simulink model "SingleTrackCANoe"  (R2021b)
settings: Solver=ode1  StartTime=0  StopTime=2  FixedStep=1.0000000000000000e-003  RelTol=1e-3
InitFcn:
  | sampleTime = str2double(get_param(bdroot, 'FixedStep'));
undefined symbols (not defined in the file or in its folder): AccPedalPos, BrakePedalPos, BrakeSwitch, DiscIntNeverNeededParam, DYNA4, EngSpd, IgnitionSwitch, InitialGear, InitialSpeed, IntendedEngTrq, LeftIndicator, MainBrakePress, MaxGear, MDL, MinGear, RefAcc, RefLane, RefLatPos, RefPath, RefPathCurv, RefSpd, RefSpdPreview, RefSpdRetrospect, RightIndicator, SteeringWheelAng, SteeringWheelTrq, UserDefinedRefValue, vm_const
libraries: UtilitiesLibrary x62, simulink x18, WheelSystemModules x14, LongitudinalControllerModules x13, LateralControllerModules x7, AnimationBusselectorModules x5, EnvironmentModules x5, BasicEngineControlModules x5, MiscellaneousControlModules x5, Animation3Modules x4, AuxiliariesModules x4, ReducedTireModules x4
(part 12 of 34)

== system SingleTrackCANoe/SimulationModel/Vehicle/Engine/EngineControlUnit ==
  fromEnginePhysics : Inport
  fromCTRL : Inport  Port=2
  fromEnvironment : Inport  Port=3
  fromChassis : Inport  Port=4
  fromDrivetrain : Inport  Port=5
  fromElectricalSystem : Inport  Port=6
  ASR/MSR : BasicEngineControlModules/ASR//MSR  SystemSampleTime=-1  VariantActivationTime=update diagram  Latency=0  AutoFrameSizeCalculation=off
  Data Type Conversion{,1..4} (5 alike) : DataTypeConversion  OutDataTypeStr=double
  DynaComponentInfo : Subsystem  Tag=DynaComponentInfo
      mask init:
      | data= get_param(gcb, 'UserData');
      settings: OpenFcn=DYNA4.ModelHandling.Component.ShowEditComponentInformationDialog(gcb);
      mask Display: disp(['Type = ', data.type, '\nGroup = ', data.group, '\nName = ', data.name ])
  EngineControlUnitOutput : Subsystem  Tag=TESIS DYNAware Interface Block  mask{NeedsUpdate=off, SignalInfo=|}
      mask SignalInfo=|
      | {
      |   "Version": "4.6",
      |   "MuxedOutputBusName": "EngineControlUnit",
      |   "MuxedInputBusName": "input",
      |   "MuxedInputSelected": false,
      |   "MuxedOutputSelected": true,
      |   "SignalData": [
      |     {
      |       "initialValue": "0.0",
      |       "name": "StarterSwitch[0;1]",
      |       "comment": "Engine starter switch",
      |       "minString": "",
      |       "maxString": "",
      |       "width": 1,
      |       "dataType": 0,
      |       "signalType": 0,
      |       "createSignal": false,
      |       "outputName": "StarterSwitch[0;1]",
      |       "generateSignalAccessBlock": false,
      |       "accessId": "$(parentId).$(blockName).$(outputName)"
      |     },
      |     {
      |       "initialValue": "0.0",
      |       "name": "EngRunPermission[0;1]",
      |       "comment": "Switch indicating a engine stop due to start stop function or ignition off",
      |       "minString": "",
      |       "maxString": "",
      |       "width": 1,
      |       "dataType": 0,
      |       "signalType": 0,
      |       "createSignal": false,
      |       "outputName": "EngRunPermission[0;1]",
      |       "generateSignalAccessBlock": false,
      |       "accessId": "$(parentId).$(blockName).$(outputName)"
      |     },
      |     {
      |       "initialValue": "0.0",
      |       "name": "EngLoadSignal[0_1]",
      |       "comment": "Engine load signal",
      |       "minString": "",
      |       "maxString": "",
      |       "width": 1,
      |       "dataType": 0,
      |       "signalType": 0,
      |       "createSignal": false,
      |       "outputName": "EngLoadSignal[0_1]",
      |       "generateSignalAccessBlock": false,
      |       "accessId": "$(parentId).$(blockName).$(outputName)"
      |     },
      |     {
      |       "initialValue": "0.0",
      |       "name": "EngIdleSpd[rad/s]",
      |       "comment": "Engine idle speed",
      |       "minString": "",
      |       "maxString": "",
      |       "width": 1,
      |       "dataType": 0,
      |       "signalType": 0,
      |       "createSignal": false,
      |       "outputName": "EngIdleSpd[rad/s]",
      |       "generateSignalAccessBlock": false,
      |       "accessId": "$(parentId).$(blockName).$(outputName)"
      |     },
      |     {
      |       "initialValue": "0.0",
      |       "name": "EngFuelCutoff[0;1]",
      |       "comment": "Logical signal which is true if fuel mass flow is stopped",
      |       "minString": "",
      |       "maxString": "",
      |       "width": 1,
      |       "dataType": 0,
      |       "signalType": 0,
      |       "createSignal": false,
      |       "outputName": "EngFuelCutoff[0;1]",
      |       "generateSignalAccessBlock": false,
      |       "accessId": "$(parentId).$(blockName).$(outputName)"
      |     },
      |     {
      |       "initialValue": "0.0",
      |       "name": "MaxEngSpd[rad/s]",
      |       "comment": "Maximum allowed engine speed, threshold for fuel cut off",
      |       "minString": "",
      |       "maxString": "",
      |       "width": 1,
      |       "dataType": 0,
      |       "signalType": 0,
      |       "createSignal": false,
      |       "outputName": "MaxEngSpd[rad/s]",
      |       "generateSignalAccessBlock": false,
      |       "accessId": "$(parentId).$(blockName).$(outputName)"
      |     },
      |     {
      |       "initialValue": "0.0",
      |       "name": "UpperEngTrqSwitch[0;2]",
      |       "comment": "Switch indicating how the upper engine torque should be restricted (0: off, 1: slow, 2: fast)",
      |       "minString": "",
      |       "maxString": "",
      |       "width": 1,
      |       "dataType": 0,
      |       "signalType": 0,
      |       "createSignal": false,
      |       "outputName": "UpperEngTrqSwitch[0;2]",
      |       "generateSignalAccessBlock": false,
      |       "accessId": "$(parentId).$(blockName).$(outputName)"
      |     },
      |     {
      |       "initialValue": "0.0",
      |       "name": "UpperEngTrqLimit[Nm]",
      |       "comment": "Upper limit for the engine torque",
      |       "minString": "",
      |       "maxString": "",
      |       "width": 1,
      |       "dataType": 0,
      |       "signalType": 0,
      |       "createSignal": false,
      |       "outputName": "UpperEngTrqLimit[Nm]",
      |       "generateSignalAccessBlock": false,
      |       "accessId": "$(parentId).$(blockName).$(outputName)"
      |     },
      |     {
      |       "initialValue": "0.0",
      |       "name": "LowerEngTrqSwitch[0;2]",
      |       "comment": "Switch indicating how the lower engine torque should be restricted (0: off, 1: slow, 2: fast)",
      |       "minString": "",
      |       "maxString": "",
      |       "width": 1,
      |       "dataType": 0,
      |       "signalType": 0,
      |       "createSignal": false,
      |       "outputName": "LowerEngTrqSwitch[0;2]",
      |       "generateSignalAccessBlock": false,
      |       "accessId": "$(parentId).$(blockName).$(outputName)"
      |     },
      |     {
      |       "initialValue": "0.0",
      |       "name": "LowerEngTrqLimit[Nm]",
      |       "comment": "Lower limit for the engine torque",
      |       "minString": "",
      |       "maxString": "",
      |       "width": 1,
      |       "dataType": 0,
      |       "signalType": 0,
      |       "createSignal": false,
      |       "outputName": "LowerEngTrqLimit[Nm]",
      |       "generateSignalAccessBlock": false,
      |       "accessId": "$(parentId).$(blockName).$(outputName)"
      |     }
      |   ]
      | }
      mask prompts: NeedsUpdate "Specify, if subsystem content needs to be updated"; SignalInfo "Signal Info (json)"
      mask help: DYNA4 Interface Block Version 4.6
      mask init:
      | blockName = get_param(gcbh, 'Name');
      | parentId = DYNA4.ModelHandling.AccessID.getFromHierarchy(gcbh);
      | TD.InterfaceBlock.ModelCallbacks.GenerateContent(gcb);
      settings: DeleteFcn=TD.InterfaceBlock.ModelCallbacks.CloseGUI( gcbh );  NameChangeFcn=TD.InterfaceBlock.ModelCallbacks.BlockRenamedHandler(gcbh);  OpenFcn=TD.InterfaceBlock.ModelCallbacks.OpenGUI( gcbh );  CloseFcn=TD.InterfaceBlock.ModelCallbacks.CloseGUI( gcbh );
      mask Display:
      | image('InterfaceBlock.png','center');
      | port_label('input',1, 'StarterSwitch[0;1]');
      | port_label('input',2, 'EngRunPermission[0;1]');
      | port_label('input',3, 'EngLoadSignal[0_1]');
      | port_label('input',4, 'EngIdleSpd[rad/s]');
      | port_label('input',5, 'EngFuelCutoff[0;1]');
      | port_label('input',6, 'MaxEngSpd[rad/s]');
      | port_label('input',7, 'UpperEngTrqSwitch[0;2]');
      | port_label('input',8, 'UpperEngTrqLimit[Nm]');
      | port_label('input',9, 'LowerEngTrqSwitch[0;2]');
      | port_label('input',10, 'LowerEngTrqLimit[Nm]');
      | port_label('output',1, 'EngineControlUnit');
  EngineStartStopLogic : BasicEngineControlModules/EngineStartStopLogic  SystemSampleTime=-1  VariantActivationTime=update diagram  Latency=0  AutoFrameSizeCalculation=off
  FuelCutoff : BasicEngineControlModules/FuelCutoff  DATA_NODE=MDL.Vehicle.Engine.EngineControlUnit.FuelCutoff  FuelCutoffTimeConst=MDL.Vehicle.Engine.EngineControlUnit.FuelCutoff.FuelCutoffTimeConst  FuelCutoffPedalMax=MDL.Vehicle.Engine.EngineControlUnit.FuelCutoff.FuelCutoffMaxLoadSig  MaxEngSpd=MDL.Vehicle.Engine.EngineControlUnit.FuelCutoff.MaxEngSpd
  IdleSpeedController : BasicEngineControlModules/IdleSpeedController  DATA_NODE=MDL.Vehicle.Engine.EngineControlUnit.IdleSpeedController  RefEngIdleSpd=MDL.Vehicle.Engine.EngineControlUnit.IdleSpeedController.RefEngIdleSpd  UpperIdleSpeedThreshold=MDL.Vehicle.Engine.EngineControlUnit.IdleSpeedController.UpperIdleSpdThres  LowerIdleSpeedThreshold=MDL.Vehicle.Engine.EngineControlUnit.IdleSpeedController.LowerIdleSpdThres  MaxCtrlTrq=MDL.Vehicle.Engine.EngineControlUnit.IdleSpeedController.MaxIdleSpdRefTrq  MinCtrlTrq=MDL.Vehicle.Engine.EngineControlUnit.IdleSpeedController.MinIdleSpdRefTrq  IdleCtl_P=MDL.Vehicle.Engine.EngineControlUnit.IdleSpeedController.ProportionalGain  IdleCtl_I=MDL.Vehicle.Engine.EngineControlUnit.IdleSpeedController.IntegralGain  IdleCtl_D=MDL.Vehicle.Engine.EngineControlUnit.IdleSpeedController.DerivativeGain  IdleCtl_N=MDL.Vehicle.Engine.EngineControlUnit.IdleSpeedController.DerivativeFilterCutoffFreq  MaxIgnitionOffsetAng=MDL.Vehicle.Engine.EngineControlUnit.IdleSpeedController.MaxIgnitionOffsetAng  IgnitionDelayReductionTrq=MDL.Vehicle.Engine.EngineControlUnit.IdleSpeedController.IgnitionDelayReductionTrq  IntendedEngineStartTime=MDL.Vehicle.Engine.EngineControlUnit.IdleSpeedController.IntendedEngineStartTime
  InputFromCTRL : Subsystem  Tag=TESIS DYNAware Interface Block  mask{NeedsUpdate=off, SignalInfo=|}
      mask SignalInfo=|
      | {
      |   "Version": "4.6",
      |   "MuxedOutputBusName": "Drivetrain",
      |   "MuxedInputBusName": "fromCTRL",
      |   "MuxedInputSelected": true,
      |   "MuxedOutputSelected": false,
      |   "SignalData": [
      |     {
      |       "initialValue": "0.0",
      |       "name": "CTRL.LongitudinalControl.IgnitionSwitch[0;3]",
      |       "comment": "Ignition signal with four signal states: 0 - ignition off + consumer off + starter off, 1 - ignition off + consumer on + starter off, 2 - ignition on + consumer on + starter off, 3 - ignition on + consumer on  + starter on",
      |       "minString": "",
      |       "maxString": "",
      |       "width": 1,
      |       "dataType": 0,
      |       "signalType": 0,
      |       "createSignal": false,
      |       "outputName": "IgnitionSwitch[0;3]",
      |       "generateSignalAccessBlock": false,
      |       "accessId": "$(parentId).$(blockName).$(outputName)"
      |     },
      |     {
      |       "initialValue": "0.0",
      |       "name": "CTRL.LongitudinalControl.EngRunPermission[0;1]",
      |       "comment": "",
      |       "minString": "",
      |       "maxString": "",
      |       "width": 1,
      |       "dataType": 0,
      |       "signalType": 0,
      |       "createSignal": false,
      |       "outputName": "EngRunPermission[0;1]",
      |       "generateSignalAccessBlock": false,
      |       "accessId": "$(parentId).$(blockName).$(outputName)"
      |     },
      |     {
      |       "initialValue": "0.0",
      |       "name": "CTRL.LongitudinalControl.AccPedalPos[0_1]",
      |       "comment": "",
      |       "minString": "",
      |       "maxString": "",
      |       "width": -1,
      |       "dataType": 0,
      |       "signalType": 0,
      |       "createSignal": false,
      |       "outputName": "AccPedalPos[0_1]",
      |       "generateSignalAccessBlock": false,
      |       "accessId": "$(parentId).$(blockName).$(outputName)"
      |     },
      |     {
      |       "initialValue": "0.0",
      |       "name": "CTRL.LongitudinalControl.IntendedEngTrq[Nm]",
      |       "comment": "",
      |       "minString": "",
      |       "maxString": "",
      |       "width": 1,
      |       "dataType": 0,
      |       "signalType": 0,
      |       "createSignal": false,
      |       "outputName": "IntendedEngTrq[Nm]",
      |       "generateSignalAccessBlock": false,
      |       "accessId": "$(parentId).$(blockName).$(outputName)"
      |     },
      |     {
      |       "initialValue": "0.0",
      |       "name": "CTRL.LongitudinalControl.IntendedEngTrqActive[0;1]",
      |       "comment": "",
      |       "minString": "",
      |       "maxString": "",
      |       "width": 1,
      |       "dataType": 0,
      |       "signalType": 0,
      |       "createSignal": false,
      |       "outputName": "IntendedEngTrqActive[0;1]",
      |       "generateSignalAccessBlock": false,
      |       "accessId": "$(parentId).$(blockName).$(outputName)"
      |     },
      |     {
      |       "initialValue": "0.0",
      |       "name": "CTRL.LongitudinalControl.ClutchPos[0_1]",
      |       "comment": "Clutch position",
      |       "minString": "",
      |       "maxString": "",
      |       "width": 1,
      |       "dataType": 0,
      |       "signalType": 0,
      |       "createSignal": false,
      |       "outputName": "ClutchPos[0_1]",
      |       "generateSignalAccessBlock": false,
      |       "accessId": "$(parentId).$(blockName).$(outputName)"
      |     }
      |   ]
      | }
      mask prompts: NeedsUpdate "Specify, if subsystem content needs to be updated"; SignalInfo "Signal Info (json)"
      mask help: DYNA4 Interface Block Version 4.6
      mask init:
      | blockName = get_param(gcbh, 'Name');
      | parentId = DYNA4.ModelHandling.AccessID.getFromHierarchy(gcbh);
      | TD.InterfaceBlock.ModelCallbacks.GenerateContent(gcb);
      settings: DeleteFcn=TD.InterfaceBlock.ModelCallbacks.CloseGUI( gcbh );  NameChangeFcn=TD.InterfaceBlock.ModelCallbacks.BlockRenamedHandler(gcbh);  OpenFcn=TD.InterfaceBlock.ModelCallbacks.OpenGUI( gcbh );  CloseFcn=TD.InterfaceBlock.ModelCallbacks.CloseGUI( gcbh );
      mask Display:
      | image('InterfaceBlock.png','center');
      | port_label('input',1, 'fromCTRL');
      | port_label('output',1, 'IgnitionSwitch[0;3]');
      | port_label('output',2, 'EngRunPermission[0;1]');
      | port_label('output',3, 'AccPedalPos[0_1]');
      | port_label('output',4, 'IntendedEngTrq[Nm]');
      | port_label('output',5, 'IntendedEngTrqActive[0;1]');
      | port_label('output',6, 'ClutchPos[0_1]');
  InputFromCTRL1 : Subsystem  Tag=TESIS DYNAware Interface Block  mask{NeedsUpdate=off, SignalInfo=|}
      mask SignalInfo=|
      | {
      |   "Version": "4.6",
      |   "MuxedOutputBusName": "Drivetrain",
      |   "MuxedInputBusName": "fromCTRL",
      |   "MuxedInputSelected": true,
      |   "MuxedOutputSelected": false,
      |   "SignalData": [
      |     {
      |       "initialValue": "0.0",
      |       "name": "CTRL.LongitudinalControl.ASRRequestSwitch[0;2]",
      |       "comment": "",
      |       "minString": "",
      |       "maxString": "",
      |       "width": -1,
      |       "dataType": 0,
      |       "signalType": 0,
      |       "createSignal": false,
      |       "outputName": "ASRRequestSwitch[0;2]",
      |       "generateSignalAccessBlock": false,
      |       "accessId": "$(parentId).$(blockName).$(outputName)"
      |     },
      |     {
      |       "initialValue": "0.0",
      |       "name": "CTRL.LongitudinalControl.ASRTrq[Nm]",
      |       "comment": "",
      |       "minString": "",
      |       "maxString": "",
      |       "width": -1,
      |       "dataType": 0,
      |       "signalType": 0,
      |       "createSignal": false,
      |       "outputName": "ASRTrq[Nm]",
      |       "generateSignalAccessBlock": false,
      |       "accessId": "$(parentId).$(blockName).$(outputName)"
      |     },
      |     {
      |       "initialValue": "0.0",
      |       "name": "CTRL.LongitudinalControl.MSRRequestSwitch[0;2]",
      |       "comment": "",
      |       "minString": "",
      |       "maxString": "",
      |       "width": -1,
      |       "dataType": 0,
      |       "signalType": 0,
      |       "createSignal": false,
      |       "outputName": "MSRRequestSwitch[0;2]",
      |       "generateSignalAccessBlock": false,
      |       "accessId": "$(parentId).$(blockName).$(outputName)"
      |     },
      |     {
      |       "initialValue": "0.0",
      |       "name": "CTRL.LongitudinalControl.MSRTrq[Nm]",
      |       "comment": "",
      |       "minString": "",
      |       "maxString": "",
      |       "width": -1,
      |       "dataType": 0,
      |       "signalType": 0,
      |       "createSignal": false,
      |       "outputName": "MSRTrq[Nm]",
      |       "generateSignalAccessBlock": false,
      |       "accessId": "$(parentId).$(blockName).$(outputName)"
      |     }
      |   ]
      | }
      mask prompts: NeedsUpdate "Specify, if subsystem content needs to be updated"; SignalInfo "Signal Info (json)"
      mask help: DYNA4 Interface Block Version 4.6
      mask init:
      | blockName = get_param(gcbh, 'Name');
      | parentId = DYNA4.ModelHandling.AccessID.getFromHierarchy(gcbh);
      | TD.InterfaceBlock.ModelCallbacks.GenerateContent(gcb);
      settings: DeleteFcn=TD.InterfaceBlock.ModelCallbacks.CloseGUI( gcbh );  NameChangeFcn=TD.InterfaceBlock.ModelCallbacks.BlockRenamedHandler(gcbh);  OpenFcn=TD.InterfaceBlock.ModelCallbacks.OpenGUI( gcbh );  CloseFcn=TD.InterfaceBlock.ModelCallbacks.CloseGUI( gcbh );
      mask Display:
      | image('InterfaceBlock.png','center');
      | port_label('input',1, 'fromCTRL');
      | port_label('output',1, 'ASRRequestSwitch[0;2]');
      | port_label('output',2, 'ASRTrq[Nm]');
      | port_label('output',3, 'MSRRequestSwitch[0;2]');
      | port_label('output',4, 'MSRTrq[Nm]');
  InputFromChassis : Subsystem  Tag=TESIS DYNAware Interface Block  mask{NeedsUpdate=off, SignalInfo=|}
      mask SignalInfo=|
      | {
      |   "Version": "4.6",
      |   "MuxedOutputBusName": "Drivetrain",
      |   "MuxedInputBusName": "fromChassis",
      |   "MuxedInputSelected": true,
      |   "MuxedOutputSelected": false,
      |   "SignalData": {
      |     "initialValue": "0.0",
      |     "name": "VehicleBody.AbsVel[m/s]",
      |     "comment": "",
      |     "minString": "",
      |     "maxString": "",
      |     "width": -1,
      |     "dataType": 0,
      |     "signalType": 0,
      |     "createSignal": false,
      |     "outputName": "AbsVel[m/s]",
      |     "generateSignalAccessBlock": false,
      |     "accessId": "$(parentId).$(blockName).$(outputName)"
      |   }
      | }
      mask prompts: NeedsUpdate "Specify, if subsystem content needs to be updated"; SignalInfo "Signal Info (json)"
      mask help: DYNA4 Interface Block Version 4.6
      mask init:
      | blockName = get_param(gcbh, 'Name');
      | parentId = DYNA4.ModelHandling.AccessID.getFromHierarchy(gcbh);
      | TD.InterfaceBlock.ModelCallbacks.GenerateContent(gcb);
      settings: DeleteFcn=TD.InterfaceBlock.ModelCallbacks.CloseGUI( gcbh );  NameChangeFcn=TD.InterfaceBlock.ModelCallbacks.BlockRenamedHandler(gcbh);  OpenFcn=TD.InterfaceBlock.ModelCallbacks.OpenGUI( gcbh );  CloseFcn=TD.InterfaceBlock.ModelCallbacks.CloseGUI( gcbh );
      mask Display:
      | image('InterfaceBlock.png','center');
      | port_label('input',1, 'fromChassis');
      | port_label('output',1, 'AbsVel[m/s]');
  InputFromDrivetrain : Subsystem  Tag=TESIS DYNAware Interface Block  mask{NeedsUpdate=off, SignalInfo=|}
      mask SignalInfo=|
      | {
      |   "Version": "4.6",
      |   "MuxedOutputBusName": "Drivetrain",
      |   "MuxedInputBusName": "fromDrivetrain",
      |   "MuxedInputSelected": true,
      |   "MuxedOutputSelected": false,
      |   "SignalData": [
      |     {
      |       "initialValue": "0.0",
      |       "name": "DrivetrainPhysics.Transmission.Gear[-4;20]",
      |       "comment": "",
      |       "minString": "",
      |       "maxString": "",
      |       "width": -1,
      |       "dataType": 0,
      |       "signalType": 0,
      |       "createSignal": false,
      |       "outputName": "Gear[-4;20]",
      |       "generateSignalAccessBlock": false,
      |       "accessId": "$(parentId).$(blockName).$(outputName)"
      |     },
      |     {
      |       "initialValue": "0.0",
      |       "name": "DrivetrainPhysics.EngSpd[rad/s]",
      |       "comment": "",
      |       "minString": "",
      |       "maxString": "",
      |       "width": -1,
      |       "dataType": 0,
      |       "signalType": 0,
      |       "createSignal": false,
      |       "outputName": "EngSpd[rad/s]",
      |       "generateSignalAccessBlock": false,
      |       "accessId": "$(parentId).$(blockName).$(outputName)"
      |     }
      |   ]
      | }
      mask prompts: NeedsUpdate "Specify, if subsystem content needs to be updated"; SignalInfo "Signal Info (json)"
      mask help: DYNA4 Interface Block Version 4.6
      mask init:
      | blockName = get_param(gcbh, 'Name');
      | parentId = DYNA4.ModelHandling.AccessID.getFromHierarchy(gcbh);
      | TD.InterfaceBlock.ModelCallbacks.GenerateContent(gcb);
      settings: DeleteFcn=TD.InterfaceBlock.ModelCallbacks.CloseGUI( gcbh );  NameChangeFcn=TD.InterfaceBlock.ModelCallbacks.BlockRenamedHandler(gcbh);  OpenFcn=TD.InterfaceBlock.ModelCallbacks.OpenGUI( gcbh );  CloseFcn=TD.InterfaceBlock.ModelCallbacks.CloseGUI( gcbh );
      mask Display:
      | image('InterfaceBlock.png','center');
      | port_label('input',1, 'fromDrivetrain');
      | port_label('output',1, 'Gear[-4;20]');
      | port_label('output',2, 'EngSpd[rad/s]');
  InputFromEnginePhysics : Subsystem  Tag=TESIS DYNAware Interface Block  mask{NeedsUpdate=off, SignalInfo=|}
      mask SignalInfo=|
      | {
      |   "Version": "4.6",
      |   "MuxedOutputBusName": "Drivetrain",
      |   "MuxedInputBusName": "fromEnginePhysics",
      |   "MuxedInputSelected": true,
      |   "MuxedOutputSelected": false,
      |   "SignalData": [
      |     {
      |       "initialValue": "0.0",
      |       "name": "Mechanics.EngTrq[Nm]",
      |       "comment": "Engine torque",
      |       "minString": "",
      |       "maxString": "",
      |       "width": 1,
      |       "dataType": 0,
      |       "signalType": 0,
      |       "createSignal": false,
      |       "outputName": "EngTrq[Nm]",
      |       "generateSignalAccessBlock": false,
      |       "accessId": "$(parentId).$(blockName).$(outputName)"
      |     },
      |     {
      |       "initialValue": "0.0",
      |       "name": "Mechanics.UnrestrictedEngTrq[Nm]",
      |       "comment": "Unrestricted engine torque",
      |       "minString": "",
      |       "maxString": "",
      |       "width": 1,
      |       "dataType": 0,
      |       "signalType": 0,
      |       "createSignal": false,
      |       "outputName": "UnrestrictedEngTrq[Nm]",
      |       "generateSignalAccessBlock": false,
      |       "accessId": "$(parentId).$(blockName).$(outputName)"
      |     },
      |     {
      |       "initialValue": "0.0",
      |       "name": "Mechanics.MeanEngFrictionTrq[Nm]",
      |       "comment": "",
      |       "minString": "",
      |       "maxString": "",
      |       "width": -1,
      |       "dataType": 0,
      |       "signalType": 0,
      |       "createSignal": false,
      |       "outputName": "MeanEngFrictionTrq[Nm]",
      |       "generateSignalAccessBlock": false,
      |       "accessId": "$(parentId).$(blockName).$(outputName)"
      |     },
      |     {
      |       "initialValue": "0.0",
      |       "name": "Mechanics.MeanEngMaxTrq[Nm]",
      |       "comment": "",
      |       "minString": "",
      |       "maxString": "",
      |       "width": -1,
      |       "dataType": 0,
      |       "signalType": 0,
      |       "createSignal": false,
      |       "outputName": "MeanEngMaxTrq[Nm]",
      |       "generateSignalAccessBlock": false,
      |       "accessId": "$(parentId).$(blockName).$(outputName)"
      |     }
      |   ]
      | }
      mask prompts: NeedsUpdate "Specify, if subsystem content needs to be updated"; SignalInfo "Signal Info (json)"
      mask help: DYNA4 Interface Block Version 4.6
      mask init:
      | blockName = get_param(gcbh, 'Name');
      | parentId = DYNA4.ModelHandling.AccessID.getFromHierarchy(gcbh);
      | TD.InterfaceBlock.ModelCallbacks.GenerateContent(gcb);
      settings: DeleteFcn=TD.InterfaceBlock.ModelCallbacks.CloseGUI( gcbh );  NameChangeFcn=TD.InterfaceBlock.ModelCallbacks.BlockRenamedHandler(gcbh);  OpenFcn=TD.InterfaceBlock.ModelCallbacks.OpenGUI( gcbh );  CloseFcn=TD.InterfaceBlock.ModelCallbacks.CloseGUI( gcbh );
      mask Display:
      | image('InterfaceBlock.png','center');
      | port_label('input',1, 'fromEnginePhysics');
      | port_label('output',1, 'EngTrq[Nm]');
      | port_label('output',2, 'UnrestrictedEngTrq[Nm]');
      | port_label('output',3, 'MeanEngFrictionTrq[Nm]');
      | port_label('output',4, 'MeanEngMaxTrq[Nm]');
  IntendedEngineLoad : BasicEngineControlModules/IntendedEngineLoad  DATA_NODE=MDL.Vehicle.Engine.EngineControlUnit.AcceleratorPedalCharacteristic  DATA_NODE2=MDL.Vehicle.Engine.EngineControlUnit.EngineLoadSignalCalculation
  Logical Operator1 : Logic  Operator=NOT  AllPortsSameDT=off  OutDataTypeStr=boolean
  Logical Operator2 : Logic  Operator=OR  AllPortsSameDT=off  OutDataTypeStr=boolean
  Memory : Memory  InheritSampleTime=on
  Product : Product
  Product1 : Product
  RefIdleSpdSwitch[0;1] : Constant  Value=0
  RefIdleSpd[rad/s] : Constant  Value=0
  RefTrq[Nm] : Constant  Value=0
  Terminator2 : Terminator
  Terminator_1 : Terminator
  Terminator_39 : Terminator
  fromCTRL1 : InportShadow  Port=2
  no fuel cutoff : Logic  Operator=NOT  AllPortsSameDT=off  OutDataTypeStr=boolean
  EngineControlUnit : Outport  VectorParamsAs1DForOutWhenUnconnected=off
  wires:
  Product1/1 -> EngineControlUnitOutput/9(LowerEngTrqSwitch[0;2]___UNIQUE_1)
  ASR/MSR/1 -> EngineControlUnitOutput/7(UpperEngTrqSwitch[0;2]___UNIQUE_1)
  FuelCutoff/3 -> Logical Operator2/2
  FuelCutoff/1 -> Logical Operator1/1, Data Type Conversion1/1, no fuel cutoff/1
  Logical Operator2/1 -> Data Type Conversion4/1
  Logical Operator1/1 -> Logical Operator2/1
  Data Type Conversion4/1 -> Product1/1
  fromCTRL1/1 -> InputFromCTRL1/1(fromCTRL)
  InputFromEnginePhysics/3(MeanEngFrictionTrq[Nm]___UNIQUE_1) -> IntendedEngineLoad/7
  Data Type Conversion3/1 -> EngineControlUnitOutput/2(EngRunPermission[0;1]___UNIQUE_1)
  FuelCutoff/2 -> EngineControlUnitOutput/6(MaxEngSpd[rad/s]___UNIQUE_1)
  InputFromCTRL/3(AccPedalPos[0_1]___UNIQUE_1) -> IntendedEngineLoad/1
  InputFromCTRL1/4(MSRTrq[Nm]___UNIQUE_1) -> ASR/MSR/7
  InputFromCTRL1/3(MSRRequestSwitch[0;2]___UNIQUE_1) -> ASR/MSR/6
  InputFromEnginePhysics/2(UnrestrictedEngTrq[Nm]___UNIQUE_1) -> ASR/MSR/3
  fromEnginePhysics/1 -> InputFromEnginePhysics/1(fromEnginePhysics)
  ASR/MSR/4 -> EngineControlUnitOutput/10(LowerEngTrqLimit[Nm]___UNIQUE_1)
  ASR/MSR/3 -> Product1/2
  ASR/MSR/2 -> EngineControlUnitOutput/8(UpperEngTrqLimit[Nm]___UNIQUE_1)
  Data Type Conversion/1 -> EngineControlUnitOutput/1(StarterSwitch[0;1]___UNIQUE_1)
  IdleSpeedController/1 -> EngineControlUnitOutput/4(EngIdleSpd[rad/s]___UNIQUE_1)
  IdleSpeedController/3 -> FuelCutoff/2, ASR/MSR/1
  InputFromCTRL1/1(ASRRequestSwitch[0;2]___UNIQUE_1) -> ASR/MSR/4
  IdleSpeedController/4 -> EngineStartStopLogic/3
  RefTrq[Nm]/1 -> IdleSpeedController/1
  InputFromChassis/1(AbsVel[m/s]___UNIQUE_1) -> FuelCutoff/6
  IdleSpeedController/5 -> Terminator2/1
  IntendedEngineLoad/1 -> Product/1, FuelCutoff/8, IdleSpeedController/5
  EngineStartStopLogic/2 -> Data Type Conversion3/1, IdleSpeedController/6, FuelCutoff/1, IntendedEngineLoad/2
  InputFromCTRL1/2(ASRTrq[Nm]___UNIQUE_1) -> ASR/MSR/5
  EngineStartStopLogic/1 -> Data Type Conversion/1
  InputFromDrivetrain/2(EngSpd[rad/s]) -> IdleSpeedController/2, FuelCutoff/7, IntendedEngineLoad/6
  IdleSpeedController/2 -> ASR/MSR/2
  RefIdleSpd[rad/s]/1 -> IdleSpeedController/3
  InputFromCTRL/6(ClutchPos[0_1]___UNIQUE_1) -> FuelCutoff/4
  InputFromCTRL/1(IgnitionSwitch[0;3]___UNIQUE_1) -> EngineStartStopLogic/1
  RefIdleSpdSwitch[0;1]/1 -> IdleSpeedController/4
  fromElectricalSystem/1 -> Terminator_39/1
  EngineControlUnitOutput/1(EngineControlUnit___UNIQUE_1) -> EngineControlUnit/1
  fromChassis/1 -> InputFromChassis/1(fromChassis)
  fromDrivetrain/1 -> InputFromDrivetrain/1(fromDrivetrain)
  fromCTRL/1 -> InputFromCTRL/1(fromCTRL)
  fromEnvironment/1 -> Terminator_1/1
  Product/1 -> EngineControlUnitOutput/3(EngLoadSignal[0_1]___UNIQUE_1)
  Data Type Conversion1/1 -> EngineControlUnitOutput/5(EngFuelCutoff[0;1]___UNIQUE_1)
  Data Type Conversion2/1 -> Product/2
  no fuel cutoff/1 -> Data Type Conversion2/1
  InputFromCTRL/4(IntendedEngTrq[Nm]___UNIQUE_1) -> IntendedEngineLoad/3
  InputFromCTRL/5(IntendedEngTrqActive[0;1]___UNIQUE_1) -> IntendedEngineLoad/4
  InputFromEnginePhysics/4(MeanEngMaxTrq[Nm]___UNIQUE_1) -> IntendedEngineLoad/8
  InputFromCTRL/2(EngRunPermission[0;1]___UNIQUE_1) -> EngineStartStopLogic/2
  InputFromEnginePhysics/1(EngTrq[Nm]___UNIQUE_1) -> Memory/1, FuelCutoff/5
  InputFromDrivetrain/1(Gear[-4;20]) -> IntendedEngineLoad/5, FuelCutoff/3
  Memory/1 -> IntendedEngineLoad/9

== system SingleTrackCANoe/SimulationModel/Vehicle/Engine/EngineOutputs ==
  EnginePhysics___UNIQUE_1 : Inport  Description=|
      | <name>EnginePhysics</name>
      | <comment></comment>
  EngineControlUnit___UNIQUE_1 : Inport  Description=|  Port=2
      | <name>EngineControlUnit</name>
      | <comment></comment>
  __TDO__Engine : BusCreator  Inputs=2
  Engine___UNIQUE_1 : Outport  Description=|  VectorParamsAs1DForOutWhenUnconnected=off
      | <name>EnginePhysics</name>
      | <comment></comment>
  wires:
  __TDO__Engine/1 -> Engine___UNIQUE_1/1  "Engine"
  EngineControlUnit___UNIQUE_1/1 -> __TDO__Engine/2  "EngineControlUnit"
  EnginePhysics___UNIQUE_1/1 -> __TDO__Engine/1  "EnginePhysics"
